simulink model "open_loop2"  (R2012b)
settings: Solver=ode3  StartTime=0.0  StopTime=t_total+50  FixedStep=0.001  RelTol=1e-3
values from neighbouring files (symbols this model uses):
  a = D/(8*(t1^2)*(n^2))    [Craneparameters.m]    (also in Craneparameters2.m = 0.428041999052; Craneparameters3.m = 0.428041999052; Craneparameters4.m = 0.5; Craneparameters5.m = 0.428041999052)
  a2 = D/(2*(4*p+1)*p*(t1^2))    [Craneparameters2.m]    (also in Craneparameters3.m = D/(2*(4*n+5)*(n+1)*(t1^2)); Craneparameters5.m = D/(2*(4*n+5)*(n+1)*(t1^2)))
  g = 9.81    [Craneparameters.m]    (also in Craneparameters2.m; Craneparameters3.m; Craneparameters4.m; Craneparameters5.m)
  l = 40    [Craneparameters.m]    (also in Craneparameters2.m; Craneparameters3.m; Craneparameters4.m; Craneparameters5.m)
  m = 67.3*10^3    (= 67300)    [Craneparameters.m]    (also in Craneparameters2.m; Craneparameters3.m; Craneparameters4.m; Craneparameters5.m)
  M = 26*10^3    (= 26000)    [Craneparameters.m]    (also in Craneparameters2.m; Craneparameters3.m; Craneparameters4.m; Craneparameters5.m)
  T = 2*pi/w    [Craneparameters.m]    (also in Craneparameters2.m; Craneparameters3.m; Craneparameters4.m; Craneparameters5.m)
  T1 = n*T    [Craneparameters.m]    (also in Craneparameters2.m; Craneparameters3.m; Craneparameters4.m = t1; Craneparameters5.m)
  T2 = n*T+t2    [Craneparameters.m]    (also in Craneparameters2.m; Craneparameters3.m = (n+1)*T; Craneparameters4.m = t1+t2; Craneparameters5.m = (n+1)*T)
  T3 = (n+1)*T+t2    [Craneparameters3.m]    (also in Craneparameters5.m)
  T4 = (n+2)*T+t2    [Craneparameters3.m]    (also in Craneparameters5.m)
  t_total = 2*n*T + t2    [Craneparameters.m]    (also in Craneparameters2.m = t_total2; Craneparameters3.m = 2*(n+1)*T + t2; Craneparameters4.m = T2+t1; Craneparameters5.m = 2*(n+1)*T + t2)
settings Model: Creator=mchusr  LastModifiedBy=mchusr

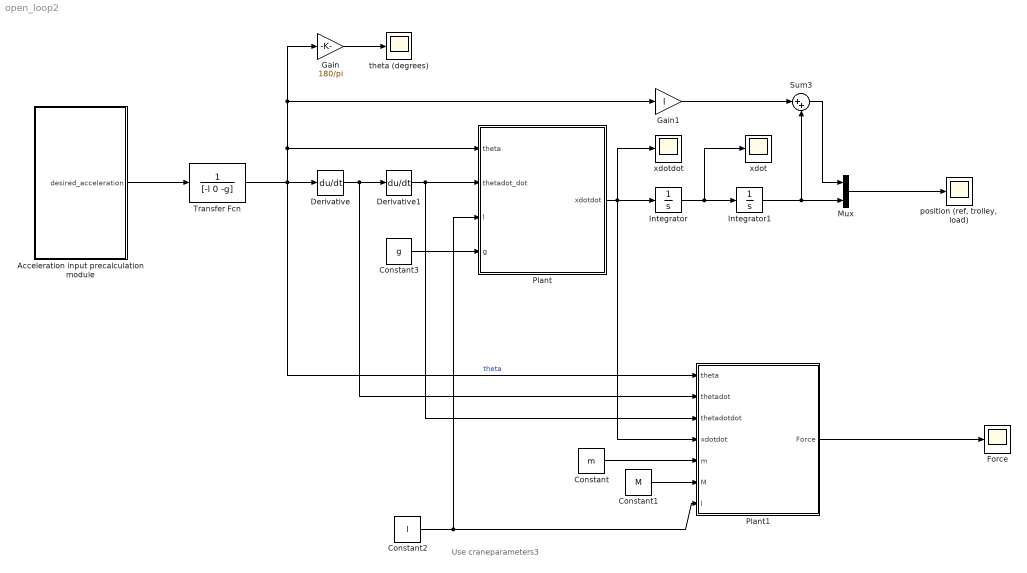
== system open_loop2 ==
  note: Use craneparameters3
  Acceleration input precalculation module : Subsystem
  Constant : Constant  Value=m
  Constant1 : Constant  Value=M
  Constant2 : Constant  Value=l
  Constant3 : Constant  Value=g
  Derivative : Derivative
  Derivative1 : Derivative
  Force : Scope
      settings: SaveName=Force
  Gain : Gain  Gain=180/pi
  Gain1 : Gain  Gain=l
  Integrator : Integrator
  Integrator1 : Integrator
  Mux : Mux  Inputs=2
  Plant : Subsystem
  Plant1 : Subsystem
  Sum3 : Sum  Inputs=|++
  Transfer Fcn : TransferFcn  Denominator=[-l 0 -g]
  "position (ref, trolley, load)" : Scope
      settings: TimeRange=120  YMin=-20  YMax=160  SaveName=position1
  theta (degrees) : Scope
      settings: SaveName=degrees
  xdot : Scope
      settings: YMin=5.55112e-17  YMax=1.9  SaveName=velocity
  xdotdot : Scope
      settings: TimeRange=105  YMin=-7.5e-08  YMax=7.5e-08  SaveName=xdotdot
  wires:
  Transfer Fcn/1 -> Gain/1, Gain1/1, Plant/1(theta), Derivative/1, Plant1/1(theta)  "theta"
  Derivative/1 -> Plant1/2(thetadot), Derivative1/1
  Derivative1/1 -> Plant1/3(thetadotdot), Plant/2(thetadot_dot)
  Plant/1(xdotdot) -> Integrator/1, Plant1/4("xdotdot "), xdotdot/1
  Plant1/1(Force) -> Force/1
  Constant1/1 -> Plant1/6(M)
  Constant/1 -> Plant1/5(m)
  Constant2/1 -> Plant/3(l), Plant1/7(l)
  Constant3/1 -> Plant/4(g)
  Integrator/1 -> xdot/1, Integrator1/1
  Integrator1/1 -> Mux/2, Sum3/2
  Gain/1 -> theta (degrees)/1
  Acceleration input precalculation module/1(desired_acceleration) -> Transfer Fcn/1
  Gain1/1 -> Sum3/1
  Mux/1 -> "position (ref, trolley, load)"/1
  Sum3/1 -> Mux/1

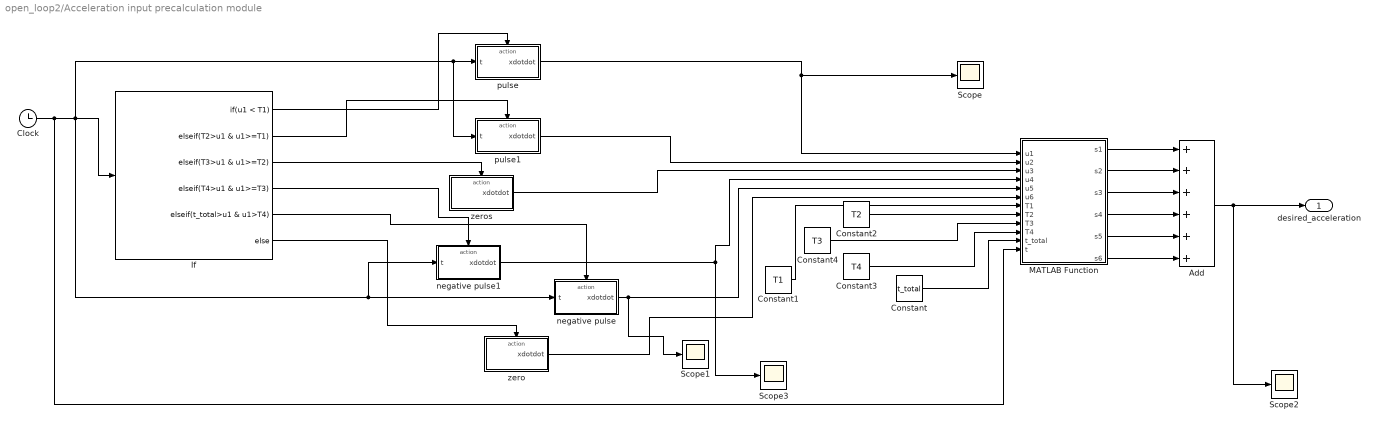
== system open_loop2/Acceleration input precalculation module ==
  Add : Sum  Inputs=++++++
  Clock : Clock
  Constant : Constant  Value=t_total
  Constant1 : Constant  Value=T1
  Constant2 : Constant  Value=T2
  Constant3 : Constant  Value=T4
  Constant4 : Constant  Value=T3
  If : If  IfExpression=u1 < T1  ElseIfExpressions=T2>u1 & u1>=T1, T3>u1 & u1>=T2, T4>u1 & u1>=T3, t_total>u1 & u1>T4  ZeroCross=off
  MATLAB Function : MATLAB Function  TreatAsAtomicUnit=on
  Scope{,1..3} (4 alike) : Scope
      Scope settings: SaveName=ScopeData4
      Scope1 settings: SaveName=ScopeData5
      Scope2 settings: SaveName=ScopeData6
  negative pulse : Subsystem  TreatAsAtomicUnit=on
  negative pulse1 : Subsystem  TreatAsAtomicUnit=on
  pulse : Subsystem  TreatAsAtomicUnit=on
  pulse1 : Subsystem  TreatAsAtomicUnit=on
  "zero " : Subsystem  TreatAsAtomicUnit=on
  zeros : Subsystem  TreatAsAtomicUnit=on
  desired_acceleration : Outport
  wires:
  If/1 -> pulse/Action
  Clock/1 -> MATLAB Function/12(t), pulse1/1(t), pulse/1(t), negative pulse1/1(t), negative pulse/1(t), If/1
  Add/1 -> Scope2/1, desired_acceleration/1
  pulse/1(xdotdot) -> MATLAB Function/1(u1), Scope/1
  MATLAB Function/1(s1) -> Add/1
  MATLAB Function/2(s2) -> Add/2
  MATLAB Function/3(s3) -> Add/3
  MATLAB Function/4(s4) -> Add/4
  Constant1/1 -> MATLAB Function/7(T1)
  Constant/1 -> MATLAB Function/11(t_total)
  MATLAB Function/5(s5) -> Add/5
  Constant2/1 -> MATLAB Function/8(T2)
  Constant4/1 -> MATLAB Function/9(T3)
  Constant3/1 -> MATLAB Function/10(T4)
  If/2 -> pulse1/Action
  pulse1/1(xdotdot) -> MATLAB Function/2(u2)
  If/3 -> zeros/Action
  zeros/1(xdotdot) -> MATLAB Function/3(u3)
  If/4 -> negative pulse1/Action
  If/5 -> negative pulse/Action
  negative pulse1/1(xdotdot) -> MATLAB Function/4(u4), Scope3/1
  negative pulse/1(xdotdot) -> Scope1/1, MATLAB Function/5(u5)
  If/6 -> "zero "/Action
  "zero "/1(xdotdot) -> MATLAB Function/6(u6)
  MATLAB Function/6(s6) -> Add/6

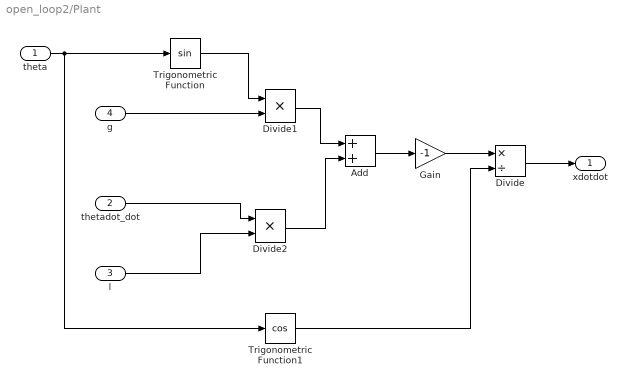
== system open_loop2/Plant ==
  theta : Inport
  thetadot_dot : Inport  Port=2
  l : Inport  Port=3
  g : Inport  Port=4
  Add : Sum
  Divide : Product  Inputs=*/
  Divide1 : Product  Inputs=**
  Divide2 : Product  Inputs=**
  Gain : Gain  Gain=-1
  Trigonometric Function : Trigonometry
  Trigonometric Function1 : Trigonometry  Operator=cos
  xdotdot : Outport
  wires:
  theta/1 -> Trigonometric Function/1, Trigonometric Function1/1
  Trigonometric Function/1 -> Divide1/1
  g/1 -> Divide1/2
  Divide1/1 -> Add/1
  thetadot_dot/1 -> Divide2/1
  l/1 -> Divide2/2
  Divide2/1 -> Add/2
  Add/1 -> Gain/1
  Gain/1 -> Divide/1
  Trigonometric Function1/1 -> Divide/2
  Divide/1 -> xdotdot/1

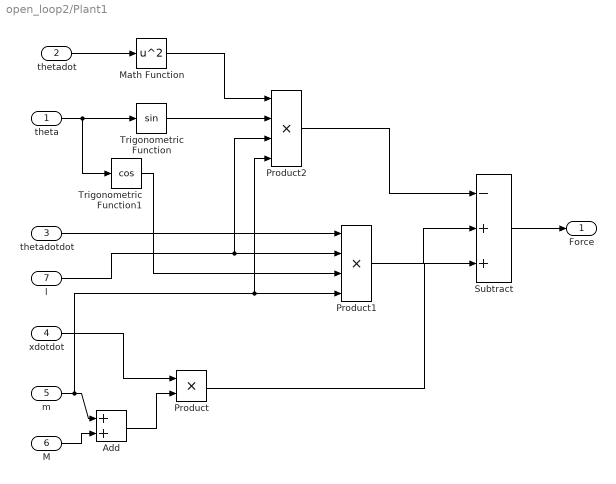
== system open_loop2/Plant1 ==
  theta : Inport
  thetadot : Inport  Port=2
  thetadotdot : Inport  Port=3
  "xdotdot " : Inport  Port=4
  m : Inport  Port=5
  M : Inport  Port=6
  l : Inport  Port=7
  Add : Sum
  Math Function : Math  Operator=square  SaturateOnIntegerOverflow=on
  Product : Product  RndMeth=Zero
  Product1 : Product  Inputs=4  RndMeth=Zero
  Product2 : Product  Inputs=4  RndMeth=Zero
  Subtract : Sum  Inputs=-++
  Trigonometric Function : Trigonometry
  Trigonometric Function1 : Trigonometry  Operator=cos
  Force : Outport
  wires:
  Subtract/1 -> Force/1
  theta/1 -> Trigonometric Function1/1, Trigonometric Function/1
  m/1 -> Product2/4, Product1/4, Add/1
  M/1 -> Add/2
  "xdotdot "/1 -> Product/1
  Add/1 -> Product/2
  thetadotdot/1 -> Product1/1
  l/1 -> Product2/3, Product1/2
  Trigonometric Function1/1 -> Product1/3
  thetadot/1 -> Math Function/1
  Math Function/1 -> Product2/1
  Trigonometric Function/1 -> Product2/2
  Product2/1 -> Subtract/1
  Product1/1 -> Subtract/2
  Product/1 -> Subtract/3

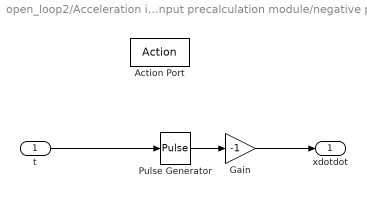
== system open_loop2/Acceleration input precalculation module/negative pulse ==
  t : Inport
  Action Port : ActionPort  ActionType=elseif
  Gain : Gain  Gain=-1
  Pulse Generator : DiscretePulseGenerator  PulseType=Time based  TimeSource=Use external signal  Amplitude=a  Period=T/2  PulseWidth=50  PhaseDelay=T4  SampleTime=0.001
  xdotdot : Outport
  wires:
  t/1 -> Pulse Generator/1
  Pulse Generator/1 -> Gain/1
  Gain/1 -> xdotdot/1

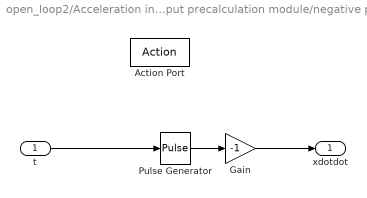
== system open_loop2/Acceleration input precalculation module/negative pulse1 ==
  t : Inport
  Action Port : ActionPort  ActionType=elseif
  Gain : Gain  Gain=-1
  Pulse Generator : DiscretePulseGenerator  PulseType=Time based  TimeSource=Use external signal  Amplitude=a2  Period=T/2  PulseWidth=50  PhaseDelay=T3  SampleTime=0.001
  xdotdot : Outport
  wires:
  t/1 -> Pulse Generator/1
  Pulse Generator/1 -> Gain/1
  Gain/1 -> xdotdot/1

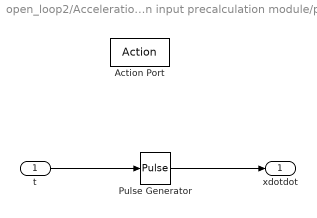
== system open_loop2/Acceleration input precalculation module/pulse ==
  t : Inport
  Action Port : ActionPort  ActionType=then
  Pulse Generator : DiscretePulseGenerator  PulseType=Time based  TimeSource=Use external signal  Amplitude=a  Period=T/2  PulseWidth=50  SampleTime=0.001
  xdotdot : Outport
  wires:
  Pulse Generator/1 -> xdotdot/1
  t/1 -> Pulse Generator/1

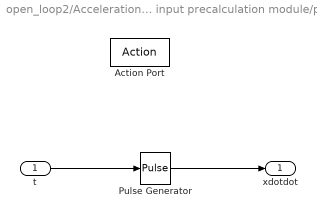
== system open_loop2/Acceleration input precalculation module/pulse1 ==
  t : Inport
  Action Port : ActionPort  ActionType=elseif
  Pulse Generator : DiscretePulseGenerator  PulseType=Time based  TimeSource=Use external signal  Amplitude=a2  Period=T/2  PulseWidth=50  PhaseDelay=T1  SampleTime=0.001
  xdotdot : Outport
  wires:
  Pulse Generator/1 -> xdotdot/1
  t/1 -> Pulse Generator/1

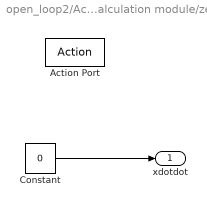
== system open_loop2/Acceleration input precalculation module/zero  ==
  Action Port : ActionPort  ActionType=else
  Constant : Constant  Value=0
  xdotdot : Outport
  wires:
  Constant/1 -> xdotdot/1

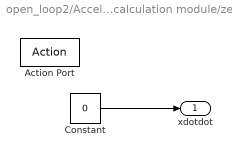
== system open_loop2/Acceleration input precalculation module/zeros ==
  Action Port : ActionPort  ActionType=elseif
  Constant : Constant  Value=0
  xdotdot : Outport
  wires:
  Constant/1 -> xdotdot/1

== matlab function open_loop2/Acceleration input precalculation module/MATLAB Function ==
  data: u1 input; s1 output; u2 input; u3 input; u4 input; u5 input; u6 input; T1 input; T2 input; T3 input; T4 input; t_total input; s2 output; s3 output; s4 output; t input; s5 output; s6 output
function [s1, s2, s3, s4, s5, s6] = filter(u1, u2, u3, u4, u5, u6, T1, T2, T3, T4, t_total, t)

if t<T1
    s1 = u1;
else
    s1=0;
end

if t<T2
    s2 = u2;
else
    s2=0;
end

s3=u3;

if t<T4
    s4 = u4;
else
    s4=0;
end

if t<t_total
    s5 = u5;
else
    s5=0;
end



s6=u6;




end
